simulink model "HandsON"  (R2023b)
settings: Solver=VariableStepAuto  StartTime=0.0  StopTime=T_stop  RelTol=1e-3
model workspace (MAT data in the model file):
  asd = 1
undefined symbols (not defined in the file): B, B_1, B_2, K, K_1, K_2, M_1, M_2
settings Model: Creator=alberto  LastModifiedBy=alberto

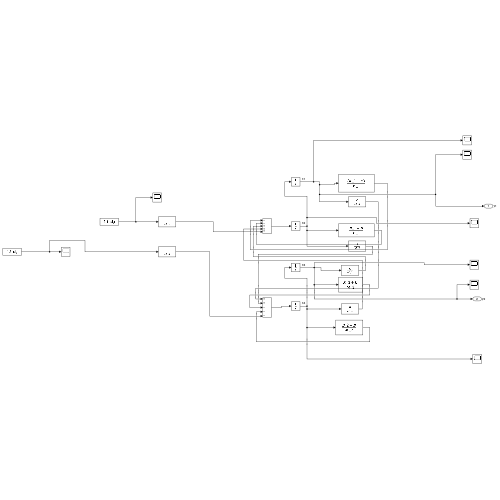
[thumbnail: Simulink's stored preview of the top-level diagram]
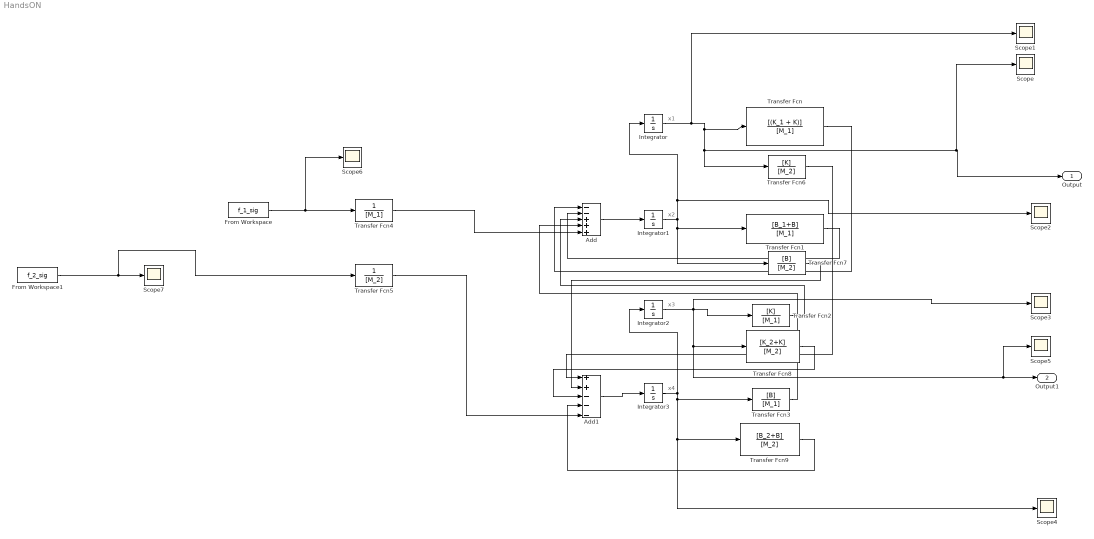
== system HandsON ==
  note: x4
  note: x3
  note: x2
  note: x1
  Add : Sum  Inputs=--+++
  Add1 : Sum  Inputs=++---
  From Workspace : FromWorkspace  VariableName=f_1_sig  OutDataTypeStr=double  SampleTime=0.01
  From Workspace1 : FromWorkspace  VariableName=f_2_sig  SampleTime=0.01
  Integrator{,1..3} (4 alike) : Integrator
  Scope{,1..7} (8 alike) : Scope
  Transfer Fcn : TransferFcn  Numerator=[(K_1 + K)]  Denominator=[M_1]
  Transfer Fcn1 : TransferFcn  Numerator=[B_1+B]  Denominator=[M_1]
  Transfer Fcn2 : TransferFcn  Numerator=[K]  Denominator=[M_1]
  Transfer Fcn3 : TransferFcn  Numerator=[B]  Denominator=[M_1]
  Transfer Fcn4 : TransferFcn  Denominator=[M_1]
  Transfer Fcn5 : TransferFcn  Denominator=[M_2]
  Transfer Fcn6 : TransferFcn  Numerator=[K]  Denominator=[M_2]
  Transfer Fcn7 : TransferFcn  Numerator=[B]  Denominator=[M_2]
  Transfer Fcn8 : TransferFcn  Numerator=[K_2+K]  Denominator=[M_2]
  Transfer Fcn9 : TransferFcn  Numerator=[B_2+B]  Denominator=[M_2]
  Output : Outport  SignalName=y1
  Output1 : Outport  Port=2  SignalName=y2
  wires:
  Integrator1/1 -> Transfer Fcn7/1, Transfer Fcn1/1, Scope2/1, Integrator/1
  Integrator3/1 -> Integrator2/1, Transfer Fcn9/1, Scope4/1, Transfer Fcn3/1
  Integrator/1 -> Scope1/1, Transfer Fcn6/1, Scope/1, Output/1, Transfer Fcn/1
  Add/1 -> Integrator1/1
  Add1/1 -> Integrator3/1
  Transfer Fcn/1 -> Add/1
  Transfer Fcn1/1 -> Add/2
  Transfer Fcn4/1 -> Add/5
  Integrator2/1 -> Scope3/1, Scope5/1, Output1/1, Transfer Fcn8/1, Transfer Fcn2/1
  Transfer Fcn2/1 -> Add/3
  Transfer Fcn3/1 -> Add/4
  Transfer Fcn6/1 -> Add1/1
  Transfer Fcn7/1 -> Add1/2
  Transfer Fcn8/1 -> Add1/3
  Transfer Fcn9/1 -> Add1/4
  Transfer Fcn5/1 -> Add1/5
  From Workspace/1 -> Transfer Fcn4/1, Scope6/1
  From Workspace1/1 -> Transfer Fcn5/1, Scope7/1
